simulink model "ETC_Model"  (R2018b)
settings: Solver=FixedStepAuto  StartTime=0.0  StopTime=Inf  FixedStep=0.001  RelTol=1e-3
PostLoadFcn:
  | if any(exist('dsrtsu_mdlpostloadfcn', 'file') ~= 0), dsrtsu_mdlpostloadfcn('Execute', bdroot); end
InitFcn:
  | , if any(exist('dsmpb_private', 'file') ~= 0), dsmpb_private('dsmpb_mdlclblib', 'Init', bdroot); end,
undefined symbols (not defined in the file): DiscIntNeverNeededParam, Gain, L, Map_Data_Values, Map_Inp_Values, Offset, R, Supply_Threshold, Theta_max, Theta_min
libraries: dsmpblib x6
PreSaveFcn:
  | , if any(exist('dsmpb_private', 'file') ~= 0), dsmpb_private('dsmpb_mdlclblib', 'PreSave', bdroot); end,
CloseFcn:
  | , if any(exist('dsmpb_private', 'file') ~= 0), dsmpb_private('dsmpb_mdlclblib', 'Close', bdroot); end,
settings Model: DSMPB_ID_DATA={'10',struct('BlockId','81d11c19-2f00-4119-8a78-f0cf1403828f','SignalIds',{{'d8e024ea-ddd4-4dd2-b0d8-d8d13ee59334'}}),'11',struct('BlockId','ed9b8333-7eb6-4c27-85fb-ebed6f81f8de','SignalIds',{{'bf70e3a8-7465-4f62-b3ea-e022f3205495'}}),'275',struct('BlockId','b7c6f48e-ff01-45b8-92e2-300eec597b54','SignalIds',{{'e94e9452-65a1-46b1-8adf-335a3f18fd66'}}),'59',struct('BlockId','bdc14eff-777a-4ffc-bf25-4fc05868bac5','SignalIds',{{'978c299e-bc19-4f18-8bd5-ea2dee079ab5'}}),'7',struct('BlockId','476f97f9-a15e-442e-86be-ad598999167e','SignalIds',{{'3cb99e27-96ec-4db8-934b-bf0a24f3002f','a2b176d5-7f95-43b9-bb17-24dc0852a657'}}),'8',struct('BlockId','5f971e07-3f4d-496b-9eb7-c98f1e8dde1c','SignalIds',{{'00d6737d-9423-4510-a55a-f7462c777906','3227f2f8-55a0-4275-b17b-3052d974dff9'}})}  RTICANMMDATA=struct('GeneralSetupData',struct('modelroot','D:\users\s003123\Desktop\Nicholas','generalsettings',struct('filesettings',struct('destfolder',struct('Name','RTICANMM_FILES','Check',1),'buildfolder',struct('Name','.','Check',1),'AbsDestfolder',struct('Name','D:\users\s003123\Desktop\Nicholas\RTICANMM_FILES'),'AbsBuildfolder',struct('Name','D:\users\s003123\Desktop\Nicholas'))),'options',struct('addpaths',1,'rmpaths',1,'addtrcexclusion',true,'cannavigator',struct('checkmonitoring',0),'show_usrtrc',0,'use_usrtrc',0),'advanced',struct('options',ones(1,100)),'MPSetup',{{}},'RTI',struct('Type','DSRT','Ver','4.2p1','Date','11-Feb-2020'),'modelname','ETC_Model','block','ETC_Model'))  DSRTSU_INTERNAL_RTIFPGA=150  Creator=S003123  LastModifiedBy=S003123
settings OptimizationCC: BlockReduction=off  ConditionallyExecuteInputs=off  OptimizeBlockIOStorage=off  BufferReuse=off  GlobalBufferReuse=off  ExpressionFolding=off  LocalBlockOutputs=off  OptimizeDataStoreBuffers=off  BusAssignmentInplaceUpdate=off
settings DebuggingCC: TasksWithSamePriorityMsg=none
settings HardwareCC: ProdBitPerPointer=32  ProdBitPerSizeT=32  ProdBitPerPtrDiffT=32  ProdLargestAtomicInteger=Integer  ProdWordSize=32  ProdHWDeviceType=Custom Processor->Custom
settings SFSimCC: MATLABDynamicMemAlloc=off
settings RTWCC: SystemTargetFile=dsrt.tlc  GenCodeOnly=on  MakeCommand=make_dsrt  TemplateMakefile=dsrt_default_tmf  Description=dSPACE Run-Time Target (for VEOS on Windows and ConfigurationDesk)  RTWVerbose=off
settings STFCustomTargetCC: TargetLangStandard=C99 (ISO)  ParMdlRefBuildCompliant=on  SystemTargetFile=dsrt.tlc
settings GRTTargetCC: CompOptLevelCompliant=off  ConcurrentExecutionCompliant=off  CombineOutputUpdateFcns=off  MatFileLogging=off  CPPClassGenCompliant=off  UseToolchainInfoCompliant=off

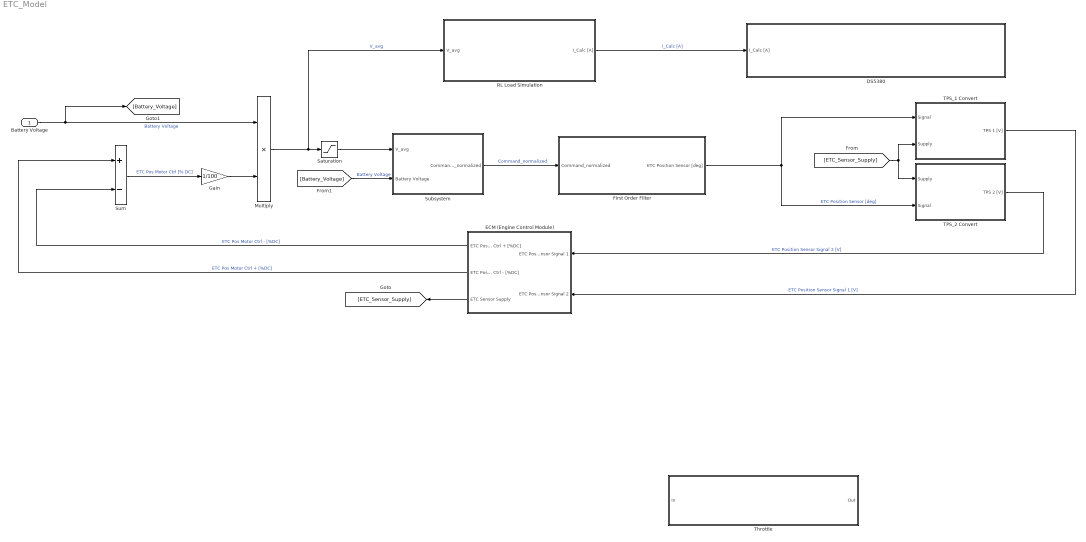
== system ETC_Model ==
  Battery Voltage : Inport
  DS5380 : Subsystem
      mask Display: image('D:\users\s003123\Desktop\Nicholas\dSPACE_logo.png');
  ECM (Engine Control Module) : Subsystem
      mask Display: image('D:\users\s003123\Desktop\Nicholas\BoschECU.png');
  "First Order Filter " : Subsystem
  Gain : Gain  Gain=1/100
  Multiply : Product
  "RL Load Simulation " : Subsystem
  Saturation : Saturate  UpperLimit=12  LowerLimit=-12
  Subsystem : Subsystem
  Sum : Sum  Inputs=+-
  TPS_1 Convert : Subsystem
  TPS_2 Convert : Subsystem
  Throttle : Subsystem  Tag=DsVdOmit=0  mask(Driveline){Block_Name=Throttle, Notes=, Application_Name=, Par_File_Name=}
      mask prompts: Block_Name "Block Name:"; Application_Name "Application Name:"; Par_File_Name "Patemeter Files:"
      mask help: Driveline Parameters
      mask init:
      | if(exist(Par_File_Name))
      |     run(Par_File_Name);
      | end
      | 
      | if(~exist('DS_CONTROLDESK_EVALUATION'))
      |    BlockParent = gcb;
      |    ModelIsStopped = 0;
      |    BlockType = '';
      |    gcb;
      | 
      |    while(~isempty(BlockParent))
      |       if(~strcmp(BlockType, 'BlockDiagram') )
      |          % get the parent block
      |          BlockParent = get_param(BlockParent, 'Parent');
      |          if(~isempty(BlockParent))
      |             % has this block another parent block
      |             if(isempty(get_param(BlockParent, 'Parent')))
      |                % no, so is is a block diagram
      |                BlockType = 'BlockDiagram';
      |             end;  % if(isempty(get_param(BlockParent, 'Parent')))
      |          end;  % if(~isempty(BlockParent))
      |       else  % if(~strcmp(BlockType, 'BlockDiagram') )
      |          if(strcmp('stopped', get_param(BlockParent, 'SimulationStatus')))
      |             ModelIsStopped = 1;
      |          end;
      |          BlockParent = '';
      |       end;  % if(~strcmp(BlockType, 'BlockDiagram') )
      |    end;  % while(~isempty(BlockParent))
      | 
      |    if(ModelIsStopped)
      |        %[X1 Y1 X2 Y2]=get_param(BlockPath,'Position')
      |        %set_param(BlockPath,'Position',[X1 Y1 X2 Y2])
      |        %[X1 Y1 X2 Y2]=get_param(BlockParent,'Position')
      |        Subsystem_Pos=get_param(gcb,'Position');
      |        Y_val=(Subsystem_Pos(4)+Subsystem_Pos(2))/2;
      |        X_val=(Subsystem_Pos(3)+Subsystem_Pos(1))/2;
      |        set_param(gcb,'Position',[X_val-175 Y_val-45 X_val+175 Y_val+45]);
      | 
      |     
      |        
      |    end;  % if(ModelIsStopped)
      | end;  % if(~exist('DS_CONTROLDESK_EVALUATION'))
      mask Help: Coast-down parameters are in [N]F0, [N*h/km]F1 e [N*h2/km2]F2.
      mask DialogControl Container3 Prompt: Icon
      mask Display:
      | % Icon Units: normalized
      | 
      | eval(strcat('text(0.25,0.75,''{\bf',Block_Name,'}'' , ''horizontalAlignment'', ''center'', ''verticalAlignment'', ''middle'',''texmode'',''on'')' ))
      | eval(strcat('text(0.25,0.62,''',Notes,''' , ''horizontalAlignment'', ''center'', ''verticalAlignment'', ''middle'',''texmode'',''on'')' ))
      | eval(strcat('text(0.25,0.45,''{\it',Application_Name,'}'' , ''horizontalAlignment'', ''center'', ''verticalAlignment'', ''middle'',''texmode'',''on'')' ))
      | 
      | port_label('Input', 1, 'In');
      | port_label('output', 1, 'Out');
      | 
      | Xgain=1.2/4500;
      | Ygain=1.2/900;
      | Xoffset=0.437;
      | Yoffset=0.52;
      | a = 0.45;
      | b = 0.93;
      | c = 0.02;
      | d = 0.8;
      | 
      | 
      | patch([a a b b a], [c d d c c],[1 1 1]);
      | plot([a a b b a], [c d d c c]);
      | 
      | text((a+b)/2, 0.28, 'S   Y   S   T   E   M   S','horizontalAlignment', 'center', 'verticalAlignment', 'middle');
      | text((a+b)/2, 0.11, 'Controls - Multi Module HIL','horizontalAlignment', 'center', 'verticalAlignment', 'middle');
      | 
      | A1 = [995 0; 1051 97; 1075 97; 1022 0; 998 0];
      | A2 = [1079 97; 1102 97; 1155 0; 1131 0; 1088 80];
      | N = [1201 97; 1224 97; 1242 82; 1260 68; 1278 54; 1296 40; 1314 26; 1316 26; 1316 97; 1338 97; 1338 0; 1315 0; 1225 71; 1223 71; 1223 0; 1201 0];
      | E=[507 98;619 98;614 84;530 84;530 56;597 56;592 42;530 42;530 14;619 14;614 0;507 0];I=[1578 97;1600 97;1600 0;1578 0];
      | L=[686 99;708 99;708 16;709 15;792 15;786 0;686 0];
      | S=[131 80;142 95;152 99;262 99;257 85;163 85;152 68;161 58;238 58;254 51;262 38;262 20;252 5;237 0;131 0;136 15;231 15;241 31;231 42;153 42;137 51;131 61];
      | T=[311 86;316 98;458 98;453 84;397 84;396 83;396 0;374 0;374 83;373 84;311 84];
      | s1=156;
      | s2=1077;
      | s3=1519;
      | 
      | S = S .* [Xgain, Ygain] + [Xoffset, Yoffset];
      | T = T .* [Xgain, Ygain] + [Xoffset, Yoffset];
      | E = E .* [Xgain, Ygain] + [Xoffset, Yoffset];
      | L = L .* [Xgain, Ygain] + [Xoffset, Yoffset];
      | A1 = A1 .* [Xgain, Ygain] + [Xoffset, Yoffset];
      | A2 = A2 .* [Xgain, Ygain] + [Xoffset, Yoffset];
      | N = N .* [Xgain, Ygain] + [Xoffset, Yoffset];
      | I = I .* [Xgain, Ygain] + [Xoffset, Yoffset];
      | s1 = s1 * Xgain;
      | s2 = s2 * Xgain;
      | s3 = s3 * Xgain;
      | 
      | color = [34, 54, 135]/255;
      | 
      | patch( S(:, 1), S(:, 2), color)
      | patch( T(:, 1), T(:, 2), color)
      | patch( E(:, 1), E(:, 2), color)
      | patch( L(:, 1), L(:, 2), color)
      | patch( L(:, 1) + s1, L(:, 2), color)
      | patch( A1(:, 1), A1(:, 2), color)
      | patch( A2(:, 1), A2(:, 2), color)
      | patch( N(:, 1), N(:, 2), color)
      | patch( T(:, 1) + s2, T(:, 2), color)
      | patch( I(:, 1), I(:, 2), color)
      | patch( S(:, 1) + s3, S(:, 2), color)
      | 
      | 
      | Xgain_=0.65/500;
      | Ygain_=0.65/100;
      | Xoffset_=0.52;
      | Yoffset_=0.18;
      | 
      | I_ = [180 26; 190 43; 198 43; 188 26; 180 26];
      | LS_ = [149 43; 157 43; 149 29; 171 29; 173 33; 163 33; 158 35; 163 42; 167 43; 184 43; 186 42; 185 39; 176 39; 178 41; 170 41; 168 37; 178 37; 182 34; 178 28; 172 26; 138 26; 149 43];
      | N_ = [218 26; 228 43; 237 43; 238 35; 244 43; 253 43; 242 26; 234 26; 232 35; 225 26; 218 26];
      | O_ = [66 39; 74 39; 69 29; 76 29; 82 41; 66 41; 72 43; 88 43; 91 42; 84 28; 77 26; 63 26; 59 28; 66 39];
      | P2_ = [93 39; 101 39; 99 35; 106 35; 110 41; 94 41; 99 43; 115 43; 118 42; 114 34; 108 31; 96 31; 93 26; 85 26; 93 39];
      | P_ = [13 42; 21 42; 18 35; 25 35; 30 43; 4 43; 10 45; 36 45; 39 44; 33 33; 28 31; 15 31; 12 26; 4 26; 13 42];
      | R_ = [31 26; 39 39; 47 39; 44 35; 52 35; 56 41; 40 41; 46 43; 62 43; 65 42; 60 34; 56 33; 58 31; 55 26; 47 26; 50 31; 42 31; 39 26; 31 26];
      | U_ = [122 43; 131 43; 122 29; 130 29; 138 43; 147 43; 137 28; 131 26; 117 26; 114 28; 122 43];
      | s_ = 133;
      | 
      | P_ = P_ .* [Xgain_, Ygain_] + [Xoffset_, Yoffset_];
      | R_ = R_ .* [Xgain_, Ygain_] + [Xoffset_, Yoffset_];
      | O_ = O_ .* [Xgain_, Ygain_] + [Xoffset_, Yoffset_];
      | P2_ = P2_ .* [Xgain_, Ygain_] + [Xoffset_, Yoffset_];
      | U_ = U_ .* [Xgain_, Ygain_] + [Xoffset_, Yoffset_];
      | LS_ = LS_ .* [Xgain_, Ygain_] + [Xoffset_, Yoffset_];
      | I_ = I_ .* [Xgain_, Ygain_] + [Xoffset_, Yoffset_];
      | N_ = N_ .* [Xgain_, Ygain_] + [Xoffset_, Yoffset_];
      | s_ = s_ .* Xgain_;
      | 
      | color2 = [0, 0, 0];
      | 
      | patch( P_(:, 1), P_(:, 2), color2)
      | patch( R_(:, 1), R_(:, 2), color2)
      | patch( O_(:, 1), O_(:, 2), color2)
      | patch( P2_(:, 1), P2_(:, 2), color2)
      | patch( U_(:, 1), U_(:, 2), color2)
      | patch( LS_(:, 1), LS_(:, 2), color2)
      | patch( I_(:, 1), I_(:, 2), color2)
      | patch( O_(:, 1) + s_, O_(:, 2), color2)
      | patch( N_(:, 1), N_(:, 2), color2)
      | 
      | % pallini
      | ox = 1077 + 0;
      | oy = 38.5 + 8;
      | 
      | ox = ox * Xgain + Xoffset;
      | oy = oy * Ygain + Yoffset ;
      | ang1 = [30 : 30 : 180 - 30] * pi / 180;
      | ang2 = [45 : 30 : 180 - 30 - 15] * pi / 180;
      | sz = [30, 20, 10] ;
      | R = [110, 130, 150];
      | alt = 0;
      | for k = 1 : length(R)
      |     if(alt == 0)
      |         %ang = [ang1, -ang1];
      |         ang = ang1;
      |         alt = 1;
      |     else
      |         %ang = [ang2, -ang2];
      |         ang = ang2;
      |         alt = 0;
      |     end
      |     for i = 1 : length(ang)
      |         x = ox + R(k) * cos(ang(i)) * Xgain;
      |         y = oy + R(k) * sin(ang(i)) * Ygain;
      |         %scatter(x, y, sz(k), color, 'filled');
      |         text(x, y, '.', 'horizontalAlignment', 'center')
      |     end
      | end
  wires:
  ECM (Engine Control Module)/2(ETC Pos Motor Ctrl - [%DC]) -> Sum/1  "ETC Pos Motor Ctrl + [%DC]"
  ECM (Engine Control Module)/1(ETC Pos Motor Ctrl + [%DC]) -> Sum/2  "ETC Pos Motor Ctrl - [%DC]"
  Sum/1 -> Gain/1  "ETC Pos Motor Ctrl [% DC]"
  Battery Voltage/1 -> [Battery_Voltage], Multiply/1  "Battery Voltage"
  TPS_1 Convert/1(TPS 1 [V]) -> ECM (Engine Control Module)/2(ETC Position Sensor Signal 2)  "ETC Position Sensor Signal 1 [V]"
  TPS_2 Convert/1(TPS 2 [V]) -> ECM (Engine Control Module)/1(ETC Position Sensor Signal 1)  "ETC Position Sensor Signal 2 [V]"
  [ETC_Sensor_Supply] -> TPS_2 Convert/1(Supply), TPS_1 Convert/2(Supply)
  ECM (Engine Control Module)/3(ETC Sensor Supply) -> [ETC_Sensor_Supply]
  Multiply/1 -> Saturation/1, "RL Load Simulation "/1(V_avg)  "V_avg"
  "RL Load Simulation "/1(I_Calc [A]) -> DS5380/1(I_Calc [A])  "I_Calc [A]"
  [Battery_Voltage] -> Subsystem/2(Battery Voltage)  "Battery Voltage"
  Saturation/1 -> Subsystem/1(V_avg)
  Gain/1 -> Multiply/2
  Subsystem/1(Command_normalized) -> "First Order Filter "/1(Command_normalized)  "Command_normalized"
  "First Order Filter "/1(ETC Position Sensor [deg]) -> TPS_2 Convert/2(Signal), TPS_1 Convert/1(Signal)  "ETC Position Sensor [deg]"

== system ETC_Model/DS5380 ==
  I_Calc [A] : Inport
  CH1 - In [Pin 9] : dsmpblib/Data Outport  Priority=-10000
      settings: SourceProductName=dSPACE Model Interface Blockset
  Constant : Constant  Value=3
  Divide : Product  Inputs=*/
  wires:
  Constant/1 -> Divide/2
  I_Calc [A]/1 -> Divide/1
  Divide/1 -> CH1 - In [Pin 9]/1  "V_DS5380 [V]"

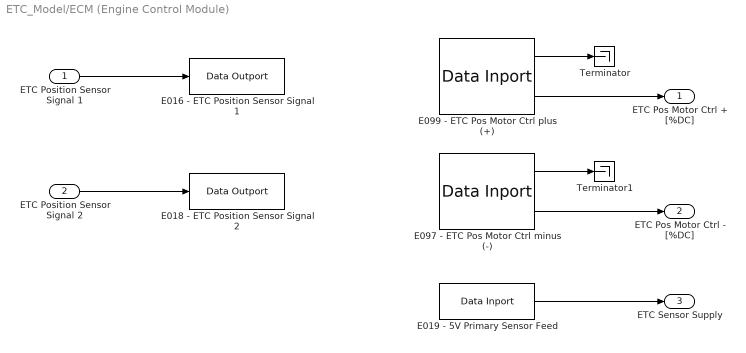
== system ETC_Model/ECM (Engine Control Module) ==
  ETC Position Sensor Signal 1 : Inport
  ETC Position Sensor Signal 2 : Inport  Port=2
  E016 - ETC Position Sensor Signal 1 : dsmpblib/Data Outport  Priority=-10000
      settings: SourceProductName=dSPACE Model Interface Blockset
  E018 - ETC Position Sensor Signal 2 : dsmpblib/Data Outport  Priority=-10000
      settings: SourceProductName=dSPACE Model Interface Blockset
  E019 - 5V Primary Sensor Feed : dsmpblib/Data Inport  Priority=10000
      settings: SourceProductName=dSPACE Model Interface Blockset
  E097 - ETC Pos Motor Ctrl minus (-) : dsmpblib/Data Inport  Priority=10000
      settings: SourceProductName=dSPACE Model Interface Blockset
  E099 - ETC Pos Motor Ctrl plus (+) : dsmpblib/Data Inport  Priority=10000
      settings: SourceProductName=dSPACE Model Interface Blockset
  Terminator : Terminator
  Terminator1 : Terminator
  ETC Pos Motor Ctrl + [%DC] : Outport
  ETC Pos Motor Ctrl - [%DC] : Outport  Port=2
  ETC Sensor Supply : Outport  Port=3
  wires:
  E099 - ETC Pos Motor Ctrl plus (+)/2 -> ETC Pos Motor Ctrl + [%DC]/1
  ETC Position Sensor Signal 1/1 -> E016 - ETC Position Sensor Signal 1/1
  ETC Position Sensor Signal 2/1 -> E018 - ETC Position Sensor Signal 2/1
  E097 - ETC Pos Motor Ctrl minus (-)/2 -> ETC Pos Motor Ctrl - [%DC]/1
  E097 - ETC Pos Motor Ctrl minus (-)/1 -> Terminator1/1
  E099 - ETC Pos Motor Ctrl plus (+)/1 -> Terminator/1
  E019 - 5V Primary Sensor Feed/1 -> ETC Sensor Supply/1

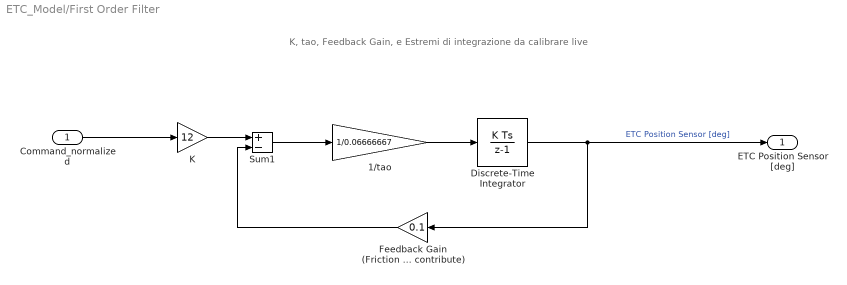
== system ETC_Model/First Order Filter  ==
  note: K, tao, Feedback Gain, e Estremi di integrazione da calibrare live
  Command_normalized : Inport
  1/tao : Gain  Gain=1/0.06666667
  Discrete-Time Integrator : DiscreteIntegrator  InitialCondition=4  SampleTime=1e-3  LimitOutput=on  UpperSaturationLimit=80  LowerSaturationLimit=2  ICPrevOutput=DiscIntNeverNeededParam  ICPrevScaledInput=DiscIntNeverNeededParam
  Feedback Gain (Friction and Elastic contribute) : Gain  Gain=0.1
  K : Gain  Gain=12
  Sum1 : Sum  Inputs=+-
  ETC Position Sensor [deg] : Outport
  wires:
  Discrete-Time Integrator/1 -> ETC Position Sensor [deg]/1, Feedback Gain (Friction and Elastic contribute)/1  "ETC Position Sensor [deg]"
  Feedback Gain (Friction and Elastic contribute)/1 -> Sum1/2
  K/1 -> Sum1/1
  Sum1/1 -> 1/tao/1
  Command_normalized/1 -> K/1
  1/tao/1 -> Discrete-Time Integrator/1

== system ETC_Model/RL Load Simulation  ==
  note: Parametri di R ed L da datasheet
  V_avg : Inport
  Gain : Gain  Gain=1/L
  Gain2 : Gain  Gain=R
  Integrator : Integrator  LimitOutput=on  UpperSaturationLimit=Theta_max  LowerSaturationLimit=Theta_min
  Sum : Sum  Inputs=+-
  I_Calc [A] : Outport
  wires:
  V_avg/1 -> Sum/1
  Gain/1 -> Integrator/1
  Integrator/1 -> Gain2/1, I_Calc [A]/1  "I_Calc [A]"
  Sum/1 -> Gain/1
  Gain2/1 -> Sum/2

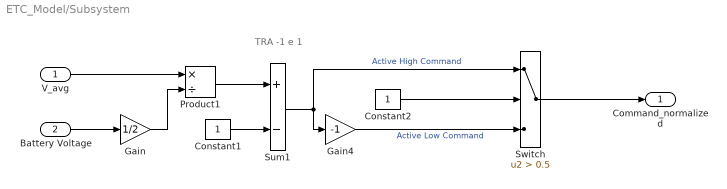
== system ETC_Model/Subsystem ==
  note: TRA -1 e 1
  V_avg : Inport
  Battery Voltage : Inport  Port=2
  Constant1 : Constant
  Constant2 : Constant
  Gain : Gain  Gain=1/2
  Gain4 : Gain  Gain=-1
  Product1 : Product  Inputs=*/
  Sum1 : Sum  Inputs=+-
  Switch : Switch  Criteria=u2 > Threshold  Threshold=0.5
  Command_normalized : Outport
  wires:
  Product1/1 -> Sum1/1
  Switch/1 -> Command_normalized/1
  V_avg/1 -> Product1/1
  Constant1/1 -> Sum1/2
  Constant2/1 -> Switch/2
  Gain4/1 -> Switch/3  "Active Low Command"
  Sum1/1 -> Gain4/1, Switch/1  "Active High Command"
  Gain/1 -> Product1/2
  Battery Voltage/1 -> Gain/1

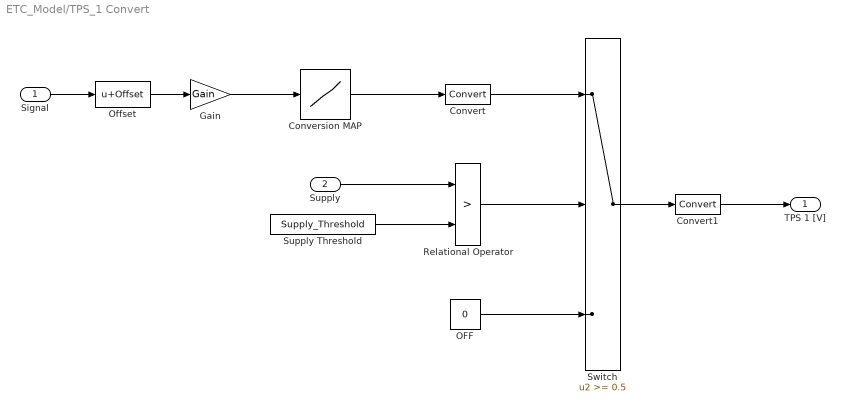
== system ETC_Model/TPS_1 Convert ==
  Signal : Inport
  Supply : Inport  Port=2
  Conversion MAP : Lookup  InputValues=Map_Inp_Values  Table=Map_Data_Values  LookUpMeth=Interpolation-Use End Values
  Convert : DataTypeConversion
  Convert1 : DataTypeConversion
  Gain : Gain  Gain=Gain
  OFF : Constant  Value=0
  Offset : Bias  Bias=Offset
  Relational Operator : RelationalOperator  Operator=>  OutDataTypeStr=boolean  RndMeth=Simplest
  Supply Threshold : Constant  Value=Supply_Threshold
  Switch : Switch  Threshold=0.5
  TPS 1 [V] : Outport
  wires:
  Conversion MAP/1 -> Convert/1
  Offset/1 -> Gain/1
  Gain/1 -> Conversion MAP/1
  Supply Threshold/1 -> Relational Operator/2
  Relational Operator/1 -> Switch/2
  OFF/1 -> Switch/3
  Switch/1 -> Convert1/1
  Supply/1 -> Relational Operator/1
  Convert/1 -> Switch/1
  Convert1/1 -> TPS 1 [V]/1
  Signal/1 -> Offset/1

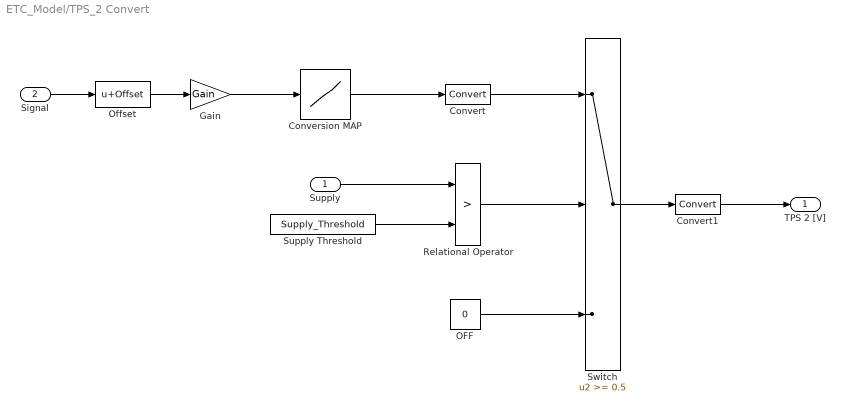
== system ETC_Model/TPS_2 Convert ==
  Supply : Inport
  Signal : Inport  Port=2
  Conversion MAP : Lookup  InputValues=Map_Inp_Values  Table=Map_Data_Values  LookUpMeth=Interpolation-Use End Values
  Convert : DataTypeConversion
  Convert1 : DataTypeConversion
  Gain : Gain  Gain=Gain
  OFF : Constant  Value=0
  Offset : Bias  Bias=Offset
  Relational Operator : RelationalOperator  Operator=>  OutDataTypeStr=boolean  RndMeth=Simplest
  Supply Threshold : Constant  Value=Supply_Threshold
  Switch : Switch  Threshold=0.5
  TPS 2 [V] : Outport
  wires:
  Signal/1 -> Offset/1
  Convert1/1 -> TPS 2 [V]/1
  Convert/1 -> Switch/1
  Supply/1 -> Relational Operator/1
  Switch/1 -> Convert1/1
  OFF/1 -> Switch/3
  Relational Operator/1 -> Switch/2
  Supply Threshold/1 -> Relational Operator/2
  Gain/1 -> Conversion MAP/1
  Offset/1 -> Gain/1
  Conversion MAP/1 -> Convert/1

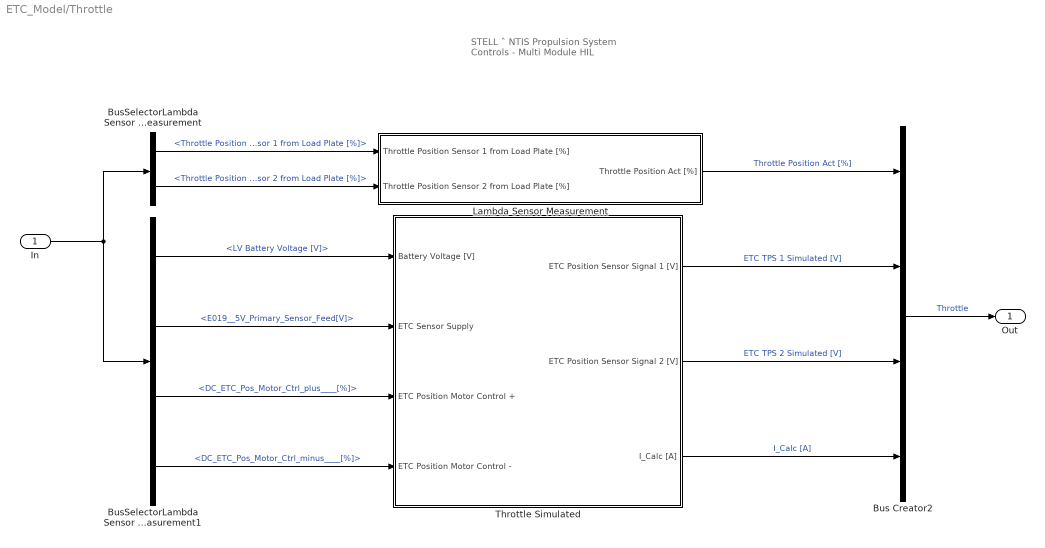
== system ETC_Model/Throttle ==
  note: STELL ˄ NTIS
      | Propulsion System
      | Controls - Multi Module HIL
  In : Inport
  Bus Creator2 : BusCreator  Inputs=4
  BusSelectorLambda Sensor Measurement : BusSelector  OutputSignals=Throttle Position Sensor 1 from Load Plate [%],Throttle Position Sensor 2 from Load Plate [%]
  BusSelectorLambda Sensor Measurement1 : BusSelector  OutputSignals=LV Battery Voltage [V],E019__5V_Primary_Sensor_Feed[V],DC_ETC_Pos_Motor_Ctrl_plus____[%],DC_ETC_Pos_Motor_Ctrl_minus____[%]
  Lambda Sensor Measurement : Subsystem
  Throttle Simulated : Subsystem
  Out : Outport
  wires:
  Lambda Sensor Measurement/1(Throttle Position Act [%]) -> Bus Creator2/1  "Throttle Position Act [%]"
  Bus Creator2/1 -> Out/1  "Throttle"
  BusSelectorLambda Sensor Measurement/1 -> Lambda Sensor Measurement/1(Throttle Position Sensor 1 from Load Plate [%])  "<Throttle Position Sensor 1 from Load Plate [%]>"
  BusSelectorLambda Sensor Measurement/2 -> Lambda Sensor Measurement/2(Throttle Position Sensor 2 from Load Plate [%])  "<Throttle Position Sensor 2 from Load Plate [%]>"
  In/1 -> BusSelectorLambda Sensor Measurement/1, BusSelectorLambda Sensor Measurement1/1
  BusSelectorLambda Sensor Measurement1/1 -> Throttle Simulated/1(Battery Voltage [V])  "<LV Battery Voltage [V]>"
  BusSelectorLambda Sensor Measurement1/2 -> Throttle Simulated/2(ETC Sensor Supply)  "<E019__5V_Primary_Sensor_Feed[V]>"
  BusSelectorLambda Sensor Measurement1/3 -> Throttle Simulated/3(ETC Position Motor Control +)  "<DC_ETC_Pos_Motor_Ctrl_plus____[%]>"
  BusSelectorLambda Sensor Measurement1/4 -> Throttle Simulated/4(ETC Position Motor Control -)  "<DC_ETC_Pos_Motor_Ctrl_minus____[%]>"
  Throttle Simulated/1(ETC Position Sensor Signal 1 [V]) -> Bus Creator2/2  "ETC TPS 1 Simulated [V]"
  Throttle Simulated/2(ETC Position Sensor Signal 2 [V]) -> Bus Creator2/3  "ETC TPS 2 Simulated [V]"
  Throttle Simulated/3(I_Calc [A]) -> Bus Creator2/4  "I_Calc [A]"

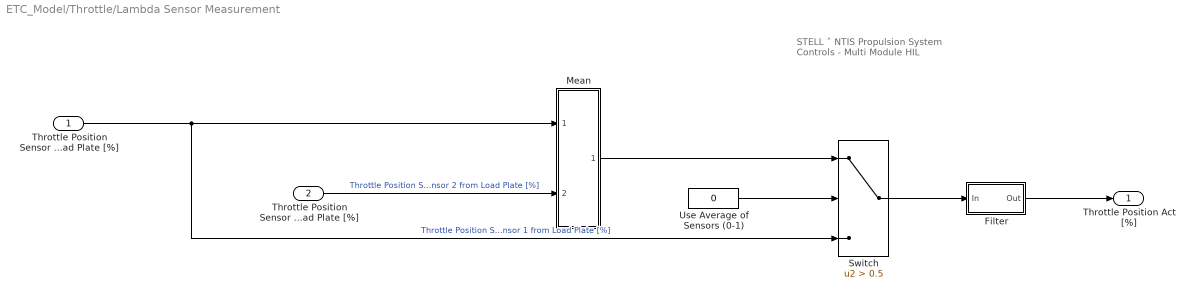
== system ETC_Model/Throttle/Lambda Sensor Measurement ==
  note: STELL ˄ NTIS
      | Propulsion System
      | Controls - Multi Module HIL
  Throttle Position Sensor 1 from Load Plate [%] : Inport
  Throttle Position Sensor 2 from Load Plate [%] : Inport  Port=2
  Filter : Subsystem  mask{tau=0.01, IC=0}
      mask prompts: tau "Time Constant [s]:"; IC "Initial Condition:"
  Mean : Subsystem
  Switch : Switch  Criteria=u2 > Threshold  Threshold=0.5
  Use Average of Sensors (0-1) : Constant  Value=0
  Throttle Position Act [%] : Outport
  wires:
  Throttle Position Sensor 1 from Load Plate [%]/1 -> Switch/3, Mean/1(In1)  "Throttle Position Sensor 1 from Load Plate [%]"
  Throttle Position Sensor 2 from Load Plate [%]/1 -> Mean/2(In2)  "Throttle Position Sensor 2 from Load Plate [%]"
  Mean/1(Out) -> Switch/1
  Filter/1(Out) -> Throttle Position Act [%]/1
  Use Average of Sensors (0-1)/1 -> Switch/2
  Switch/1 -> Filter/1(In)

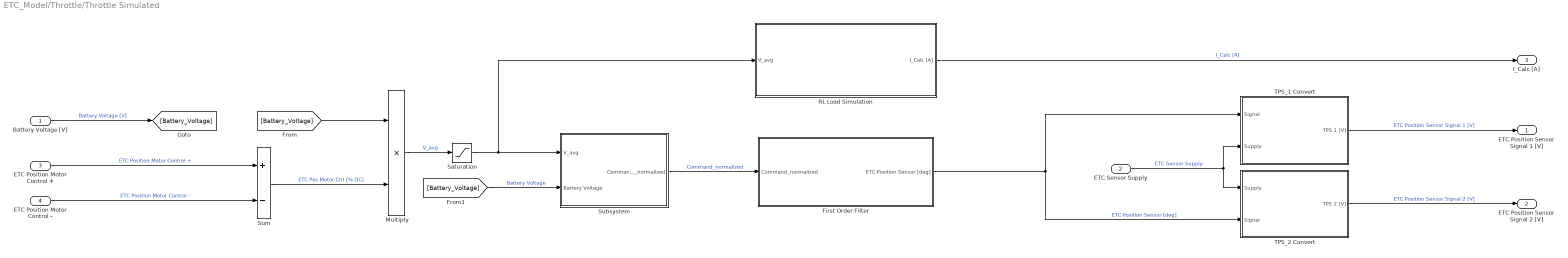
== system ETC_Model/Throttle/Throttle Simulated ==
  Battery Voltage [V] : Inport
  ETC Sensor Supply : Inport  Port=2
  ETC Position Motor Control + : Inport  Port=3
  ETC Position Motor Control - : Inport  Port=4
  "First Order Filter " : Subsystem
  Multiply : Product
  "RL Load Simulation " : Subsystem
  Saturation : Saturate  UpperLimit=12  LowerLimit=0
  Subsystem : Subsystem
  Sum : Sum  Inputs=+-
  TPS_1 Convert : Subsystem
  TPS_2 Convert : Subsystem
  ETC Position Sensor Signal 1 [V] : Outport
  ETC Position Sensor Signal 2 [V] : Outport  Port=2
  I_Calc [A] : Outport  Port=3
  wires:
  "First Order Filter "/1(ETC Position Sensor [deg]) -> TPS_1 Convert/1(Signal), TPS_2 Convert/2(Signal)  "ETC Position Sensor [deg]"
  Sum/1 -> Multiply/2  "ETC Pos Motor Ctrl [% DC]"
  TPS_1 Convert/1(TPS 1 [V]) -> ETC Position Sensor Signal 1 [V]/1  "ETC Position Sensor Signal 1 [V]"
  TPS_2 Convert/1(TPS 2 [V]) -> ETC Position Sensor Signal 2 [V]/1  "ETC Position Sensor Signal 2 [V]"
  ETC Sensor Supply/1 -> TPS_2 Convert/1(Supply), TPS_1 Convert/2(Supply)  "ETC Sensor Supply"
  ETC Position Motor Control +/1 -> Sum/1  "ETC Position Motor Control +"
  ETC Position Motor Control -/1 -> Sum/2  "ETC Position Motor Control -"
  Battery Voltage [V]/1 -> [Battery_Voltage]  "Battery Voltage [V]"
  [Battery_Voltage] -> Multiply/1
  Saturation/1 -> "RL Load Simulation "/1(V_avg), Subsystem/1(V_avg)
  [Battery_Voltage] -> Subsystem/2(Battery Voltage)  "Battery Voltage"
  Subsystem/1(Command_normalized) -> "First Order Filter "/1(Command_normalized)  "Command_normalized"
  Multiply/1 -> Saturation/1  "V_avg"
  "RL Load Simulation "/1(I_Calc [A]) -> I_Calc [A]/1  "I_Calc [A]"

== system ETC_Model/Throttle/Lambda Sensor Measurement/Filter ==
  In : Inport
  Discrete-Time Integrator : DiscreteIntegrator  InitialCondition=IC  SampleTime=-1  ICPrevOutput=DiscIntNeverNeededParam  ICPrevScaledInput=DiscIntNeverNeededParam
  Gain : Gain  Gain=1/tau  SaturateOnIntegerOverflow=on  OutDataTypeStr=Inherit: Same as input  ParamDataTypeStr=Inherit: Same as input
  Sum : Sum  Inputs=+-  SaturateOnIntegerOverflow=on  InputSameDT=on  OutDataTypeStr=Inherit: Same as first input
  Out : Outport
  wires:
  Sum/1 -> Gain/1
  Gain/1 -> Discrete-Time Integrator/1
  Discrete-Time Integrator/1 -> Sum/2, Out/1
  In/1 -> Sum/1

== system ETC_Model/Throttle/Lambda Sensor Measurement/Mean ==
  In1 : Inport
  In2 : Inport  Port=2
  Add : Sum
  Gain : Gain  Gain=0.5
  Out : Outport
  wires:
  Gain/1 -> Out/1
  Add/1 -> Gain/1
  In1/1 -> Add/1
  In2/1 -> Add/2

== system ETC_Model/Throttle/Throttle Simulated/First Order Filter  ==
  note: K, tao, Feedback Gain, e Estremi di integrazione da calibrare live
  Command_normalized : Inport
  1/tao : Gain  Gain=1/0.005
  Feedback Gain (Friction and Elastic contribute) : Gain  Gain=0.2
  Integrator : Integrator  InitialCondition=3  LimitOutput=on  UpperSaturationLimit=88  LowerSaturationLimit=2
  K : Gain  Gain=25
  Sum1 : Sum  Inputs=+-
  ETC Position Sensor [deg] : Outport
  wires:
  Sum1/1 -> 1/tao/1
  Integrator/1 -> ETC Position Sensor [deg]/1, Feedback Gain (Friction and Elastic contribute)/1  "ETC Position Sensor [deg]"
  K/1 -> Sum1/1
  1/tao/1 -> Integrator/1
  Command_normalized/1 -> K/1
  Feedback Gain (Friction and Elastic contribute)/1 -> Sum1/2

== system ETC_Model/Throttle/Throttle Simulated/RL Load Simulation  ==
  note: Parametri di R ed L da datasheet
  V_avg : Inport
  Gain : Gain  Gain=1/L
  Gain2 : Gain  Gain=R
  Integrator : Integrator  LimitOutput=on  UpperSaturationLimit=Theta_max  LowerSaturationLimit=Theta_min
  Sum : Sum  Inputs=+-
  I_Calc [A] : Outport
  wires:
  V_avg/1 -> Sum/1
  Gain/1 -> Integrator/1
  Integrator/1 -> Gain2/1, I_Calc [A]/1  "I_Calc [A]"
  Sum/1 -> Gain/1
  Gain2/1 -> Sum/2

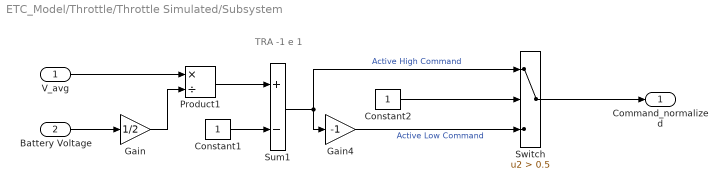
== system ETC_Model/Throttle/Throttle Simulated/Subsystem ==
  note: TRA -1 e 1
  V_avg : Inport
  Battery Voltage : Inport  Port=2
  Constant1 : Constant
  Constant2 : Constant
  Gain : Gain  Gain=1/2
  Gain4 : Gain  Gain=-1
  Product1 : Product  Inputs=*/
  Sum1 : Sum  Inputs=+-
  Switch : Switch  Criteria=u2 > Threshold  Threshold=0.5
  Command_normalized : Outport
  wires:
  Product1/1 -> Sum1/1
  Switch/1 -> Command_normalized/1
  V_avg/1 -> Product1/1
  Constant1/1 -> Sum1/2
  Constant2/1 -> Switch/2
  Gain4/1 -> Switch/3  "Active Low Command"
  Sum1/1 -> Gain4/1, Switch/1  "Active High Command"
  Gain/1 -> Product1/2
  Battery Voltage/1 -> Gain/1

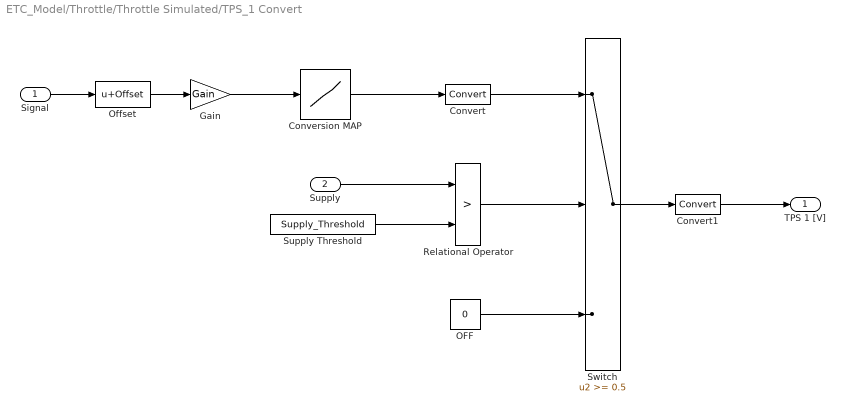
== system ETC_Model/Throttle/Throttle Simulated/TPS_1 Convert ==
  Signal : Inport
  Supply : Inport  Port=2
  Conversion MAP : Lookup  InputValues=Map_Inp_Values  Table=Map_Data_Values  LookUpMeth=Interpolation-Use End Values
  Convert : DataTypeConversion
  Convert1 : DataTypeConversion
  Gain : Gain  Gain=Gain
  OFF : Constant  Value=0
  Offset : Bias  Bias=Offset
  Relational Operator : RelationalOperator  Operator=>  OutDataTypeStr=boolean  RndMeth=Simplest
  Supply Threshold : Constant  Value=Supply_Threshold
  Switch : Switch  Threshold=0.5
  TPS 1 [V] : Outport
  wires:
  Conversion MAP/1 -> Convert/1
  Offset/1 -> Gain/1
  Gain/1 -> Conversion MAP/1
  Supply Threshold/1 -> Relational Operator/2
  Relational Operator/1 -> Switch/2
  OFF/1 -> Switch/3
  Switch/1 -> Convert1/1
  Supply/1 -> Relational Operator/1
  Convert/1 -> Switch/1
  Convert1/1 -> TPS 1 [V]/1
  Signal/1 -> Offset/1

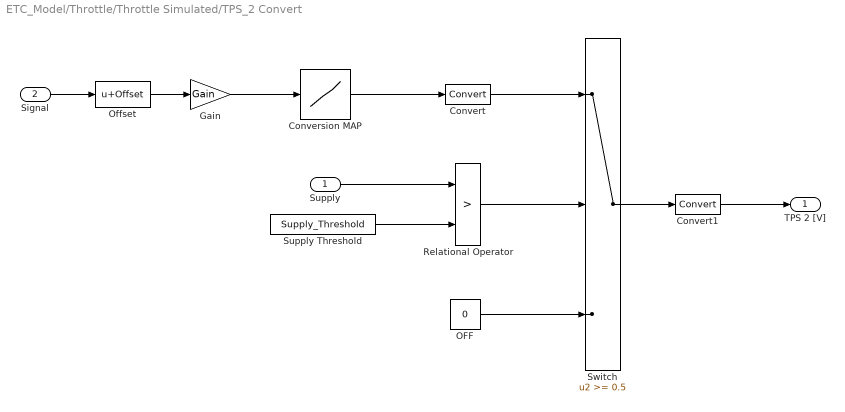
== system ETC_Model/Throttle/Throttle Simulated/TPS_2 Convert ==
  Supply : Inport
  Signal : Inport  Port=2
  Conversion MAP : Lookup  InputValues=Map_Inp_Values  Table=Map_Data_Values  LookUpMeth=Interpolation-Use End Values
  Convert : DataTypeConversion
  Convert1 : DataTypeConversion
  Gain : Gain  Gain=Gain
  OFF : Constant  Value=0
  Offset : Bias  Bias=Offset
  Relational Operator : RelationalOperator  Operator=>  OutDataTypeStr=boolean  RndMeth=Simplest
  Supply Threshold : Constant  Value=Supply_Threshold
  Switch : Switch  Threshold=0.5
  TPS 2 [V] : Outport
  wires:
  Signal/1 -> Offset/1
  Convert1/1 -> TPS 2 [V]/1
  Convert/1 -> Switch/1
  Supply/1 -> Relational Operator/1
  Switch/1 -> Convert1/1
  OFF/1 -> Switch/3
  Relational Operator/1 -> Switch/2
  Supply Threshold/1 -> Relational Operator/2
  Gain/1 -> Conversion MAP/1
  Offset/1 -> Gain/1
  Conversion MAP/1 -> Convert/1
